simulink model "sys_model"  (R2020b)
settings: Solver=VariableStepAuto  StartTime=0.0  StopTime=10.0  RelTol=1e-3
values from neighbouring files (symbols this model uses):
  C = 10    [init.m]    (also in sys_init.m = 1e-05)
  R = 10    [init.m]    (also in sys_init.m)
settings Model: Creator=Rushikesh  LastModifiedBy=Rushikesh

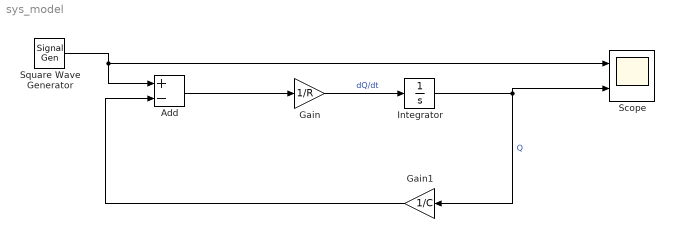
== system sys_model ==
  Add : Sum  Inputs=+-
  Gain : Gain  Gain=1/R
  Gain1 : Gain  Gain=1/C
  Integrator : Integrator  InitialCondition=0.5
  Scope : Scope  NumInputPorts=2
  Square Wave Generator : SignalGenerator  Units=rad/sec
  wires:
  Add/1 -> Gain/1
  Integrator/1 -> Gain1/1, Scope/2  "Q"
  Square Wave Generator/1 -> Add/1, Scope/1
  Gain1/1 -> Add/2
  Gain/1 -> Integrator/1  "dQ/dt"
